simulink model "buckConverter"  (R2023a)
settings: Solver=VariableStepAuto  StartTime=0.0  StopTime=inf  RelTol=1e-3
model workspace (MAT data in the model file):
  C = Simulink.Parameter
  C.Value = 0.01
  C.DataType = 'double'
  C.Complexity = 'real'
  C.Dimensions = [1 1]
  L = Simulink.Parameter
  L.Value = 0.01
  L.DataType = 'double'
  L.Complexity = 'real'
  L.Dimensions = [1 1]
  R = Simulink.Parameter
  R.Value = 10
  R.DataType = 'double'
  R.Complexity = 'real'
  R.Dimensions = [1 1]
  Vin = Simulink.Parameter
  Vin.Value = 100
  Vin.DataType = 'double'
  Vin.Complexity = 'real'
  Vin.Dimensions = [1 1]
libraries: spsCurrentMeasurementLib x8, spsSeriesRLCBranchLib x6, spsVoltageMeasurementLib x4, spsMeanLib x3, spsMosfetLib x3, spsDCVoltageSourceLib x2, spsDiodeLib x1, spspowerguiLib x1
settings Model: Creator=User  LastModifiedBy=User
settings DebuggingCC: UnconnectedInputMsg=warning  UnconnectedOutputMsg=warning  UnconnectedLineMsg=warning
settings ModelReferenceCC: EnableRefExpFcnMdlSchedulingChecks=on
settings RTWCC: DLArmComputeVersion=19.05

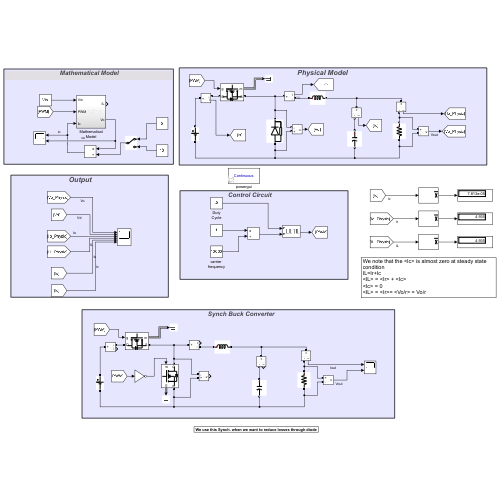
[thumbnail: Simulink's stored preview of the top-level diagram]
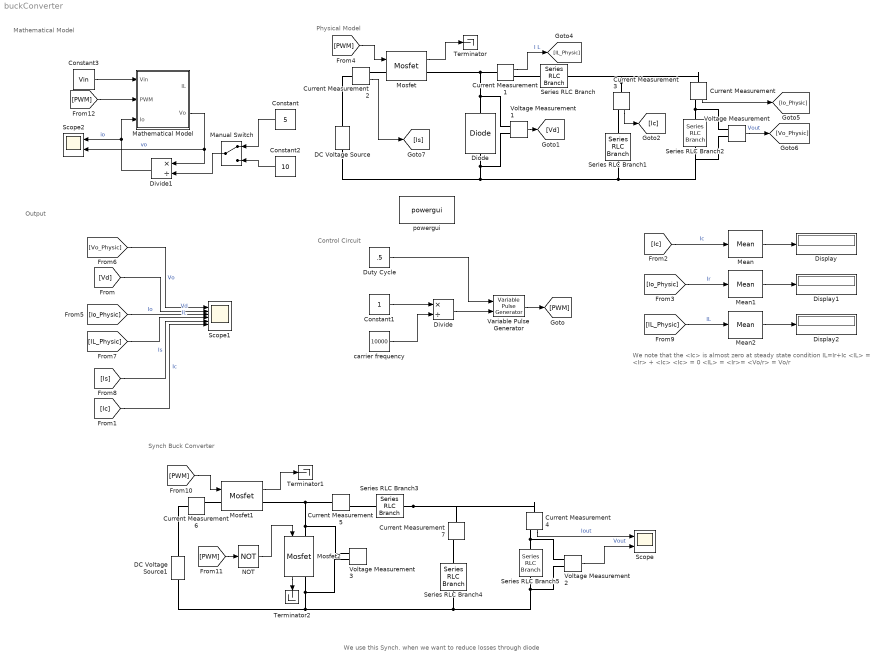
== system buckConverter ==
  note: We use this Synch. when we want to reduce losses through diode
  note: Synch Buck Converter
  note: We note that the <Ic> is almost zero at steady state condition
      | IL=Ir+Ic
      | <IL> = <Ir> + <Ic>
      | <Ic> = 0
      | <IL> = <Ir>= <Vo/r> = Vo/r
  note: Output
  note: Mathematical Model
  note: Physical Model
  note: Control Circuit
  Constant : Constant  Value=5
  Constant1 : Constant
  Constant2 : Constant  Value=10
  Constant3 : Constant  Value=Vin
  Current Measurement{,1..7} (8 alike) : spsCurrentMeasurementLib/Current Measurement  PhasorSimulation=off  OutputType=Complex  PSBequivalent=0
  DC Voltage Source : spsDCVoltageSourceLib/DC Voltage Source  Amplitude=Vin  Measurements=None
  DC Voltage Source1 : spsDCVoltageSourceLib/DC Voltage Source  Amplitude=Vin  Measurements=None
  Diode : spsDiodeLib/Diode  Ron=0.001  Lon=0  Vf=0.8  IC=0  UseSnubber=0  Rs=500  Cs=250e-9  Measurements=off
  Display : Display
  Display1 : Display
  Display2 : Display
  Divide : Product  Inputs=*/
  Divide1 : Product  Inputs=*/
  Duty Cycle : Constant  Value=.5
  Manual Switch : ManualSwitch
  Mathematical Model : Subsystem
  Mean : spsMeanLib/Mean  Freq=60  Vinit=0  Ts=0
  Mean1 : spsMeanLib/Mean  Freq=60  Vinit=0  Ts=0
  Mean2 : spsMeanLib/Mean  Freq=60  Vinit=0  Ts=0
  Mosfet : spsMosfetLib/Mosfet  Ron=0.1  Lon=0  Rd=0.01  Vfd=0  IC=0  Rs=1e5  Cs=inf  Measurements=on
  Mosfet1 : spsMosfetLib/Mosfet  Ron=0.1  Lon=0  Rd=0.01  Vfd=0  IC=0  Rs=1e5  Cs=inf  Measurements=on
  Mosfet2 : spsMosfetLib/Mosfet  Ron=0.1  Lon=0  Rd=0.01  Vfd=0  IC=0  Rs=1e5  Cs=inf  Measurements=on
  NOT : Logic  Operator=NOT  IconShape=distinctive  AllPortsSameDT=off  OutDataTypeStr=boolean
  Scope : Scope  NumInputPorts=2
  Scope1 : Scope  NumInputPorts=6
  Scope2 : Scope  NumInputPorts=2
  Series RLC Branch : spsSeriesRLCBranchLib/Series RLC Branch  LConnTagsString=__new0  RConnTagsString=__new0  BranchType=L  Resistance=1  Inductance=L  SetiL0=off  InitialCurrent=0  Capacitance=1e-6  Setx0=off  InitialVoltage=0  Measurements=None
  Series RLC Branch1 : spsSeriesRLCBranchLib/Series RLC Branch  LConnTagsString=__new0  RConnTagsString=__new0  BranchType=C  Resistance=1  Inductance=1e-3  SetiL0=off  InitialCurrent=0  Capacitance=C  Setx0=off  InitialVoltage=0  Measurements=None
  Series RLC Branch2 : spsSeriesRLCBranchLib/Series RLC Branch  LConnTagsString=__new0  RConnTagsString=__new0  BranchType=R  Resistance=R  Inductance=1e-3  SetiL0=off  InitialCurrent=0  Capacitance=1e-6  Setx0=off  InitialVoltage=0  Measurements=None
  Series RLC Branch3 : spsSeriesRLCBranchLib/Series RLC Branch  LConnTagsString=__new0  RConnTagsString=__new0  BranchType=L  Resistance=1  Inductance=L  SetiL0=off  InitialCurrent=0  Capacitance=1e-6  Setx0=off  InitialVoltage=0  Measurements=None
  Series RLC Branch4 : spsSeriesRLCBranchLib/Series RLC Branch  LConnTagsString=__new0  RConnTagsString=__new0  BranchType=C  Resistance=1  Inductance=1e-3  SetiL0=off  InitialCurrent=0  Capacitance=C  Setx0=off  InitialVoltage=0  Measurements=None
  Series RLC Branch5 : spsSeriesRLCBranchLib/Series RLC Branch  LConnTagsString=__new0  RConnTagsString=__new0  BranchType=R  Resistance=R  Inductance=1e-3  SetiL0=off  InitialCurrent=0  Capacitance=1e-6  Setx0=off  InitialVoltage=0  Measurements=None
  Terminator : Terminator
  Terminator1 : Terminator
  Terminator2 : Terminator
  Variable Pulse Generator : VariablePulseGenerator  SampleTime=0.1
  Voltage Measurement{,1..3} (4 alike) : spsVoltageMeasurementLib/Voltage Measurement  PhasorSimulation=off  OutputType=Complex  PSBequivalent=0
  carrier frequency : Constant  Value=10000
  powergui : spspowerguiLib/powergui  Priority=1  SimulationMode=Continuous  SampleTime=50e-6  frequency=60  Iterations=50  frequencyindice=0  Pbase=100e6  ErrMax=1e-4  UnitsV=kV  UnitsW=MW  buscounter=0  FunctionMessages=off  echomessages=off  EnableUseOfTLC=off  CurrentSourceSwitches=off  DisableSnubberDevices=off  DisableRonSwitches=off  DisableVfSwitches=off  DisplayEquations=off  AutomaticDiscreteSolvers=off  SolverType=Tustin/Backward Euler (TBE)  Interpol=off  ExternalGateDelay=off  methode=off  Ts=100  x0status=blocks  SPID=on  SwTol=0  HookPort=off  NonlinearTolerance=1e-4  nMaxIteration=100  ContinueOnMaxIteration=off  RestoreLinks=warning  ResistiveCurrentMeasurement=off  Frange=[0:2:500]  Ylog=off  Xlog=on  ShowGrid=off  save=off  variable=ZData  structure=0  ZoomFFT=off  StartTime=0.0  cycles=1  DisplayStyle=1  fundamental=60  FreqAxis=off  MaxFrequency=1000  frequencyindicesteady=1  RmsSteady=1  display=off
  wires:
  Variable Pulse Generator/1 -> [PWM]
  Duty Cycle/1 -> Variable Pulse Generator/1
  Divide/1 -> Variable Pulse Generator/2
  Constant1/1 -> Divide/1
  carrier frequency/1 -> Divide/2
  Mathematical Model/2(Vo) -> Divide1/1, Scope2/2  "vo"
  Divide1/1 -> Mathematical Model/3(Io), Scope2/1  "io"
  [Io_Physic] -> Scope1/3  "Io"
  [IL_Physic] -> Scope1/4  "IL"
  Current Measurement1/1 -> [IL_Physic]  "I L"
  Current Measurement/1 -> [Io_Physic]
  Voltage Measurement/1 -> [Vo_Physic]  "Vout"
  [Vo_Physic] -> Scope1/1  "Vo"
  [PWM] -> Mosfet/1
  Mosfet/1 -> Terminator/1
  Current Measurement2/1 -> [Is]
  [Is] -> Scope1/5  "Is"
  Voltage Measurement1/1 -> [Vd]
  [Vd] -> Scope1/2  "Vd"
  Current Measurement3/1 -> [Ic]
  [Ic] -> Scope1/6  "Ic"
  Mean/1 -> Display/1
  [Ic] -> Mean/1  "Ic"
  [Io_Physic] -> Mean1/1  "Ir"
  Mean1/1 -> Display1/1
  Mean2/1 -> Display2/1
  [IL_Physic] -> Mean2/1  "IL"
  Mosfet1/1 -> Terminator1/1
  [PWM] -> Mosfet1/1
  Voltage Measurement2/1 -> Scope/2  "Vout"
  Current Measurement4/1 -> Scope/1  "Iout"
  [PWM] -> NOT/1
  NOT/1 -> Mosfet2/1
  Mosfet2/1 -> Terminator2/1
  Constant/1 -> Manual Switch/1
  Manual Switch/1 -> Divide1/2
  Constant2/1 -> Manual Switch/2
  Constant3/1 -> Mathematical Model/1(Vin)
  [PWM] -> Mathematical Model/2(PWM)
  connections:
  DC Voltage Source/LConn1 -- Voltage Measurement/LConn2 -- Series RLC Branch2/RConn1 -- Series RLC Branch1/RConn1 -- Voltage Measurement1/LConn1 -- Diode/LConn1
  Series RLC Branch2/LConn1 -- Voltage Measurement/LConn1 -- Current Measurement/RConn1
  Series RLC Branch1/LConn1 -- Current Measurement3/RConn1
  Series RLC Branch/LConn1 -- Current Measurement1/RConn1
  Diode/RConn1 -- Voltage Measurement1/LConn2 -- Mosfet/RConn1 -- Current Measurement1/LConn1
  Current Measurement2/LConn1 -- DC Voltage Source/RConn1
  Mosfet/LConn1 -- Current Measurement2/RConn1
  Current Measurement3/LConn1 -- Series RLC Branch/RConn1 -- Current Measurement/LConn1
  Voltage Measurement2/LConn2 -- Series RLC Branch5/RConn1 -- Series RLC Branch4/RConn1 -- DC Voltage Source1/LConn1 -- Voltage Measurement3/LConn1 -- Mosfet2/RConn1
  Series RLC Branch5/LConn1 -- Current Measurement4/RConn1 -- Voltage Measurement2/LConn1
  Voltage Measurement3/LConn2 -- Current Measurement5/LConn1 -- Mosfet1/RConn1 -- Mosfet2/LConn1
  Series RLC Branch3/RConn1 -- Current Measurement7/LConn1 -- Current Measurement4/LConn1
  Mosfet1/LConn1 -- Current Measurement6/RConn1
  Series RLC Branch3/LConn1 -- Current Measurement5/RConn1
  Series RLC Branch4/LConn1 -- Current Measurement7/RConn1
  Current Measurement6/LConn1 -- DC Voltage Source1/RConn1

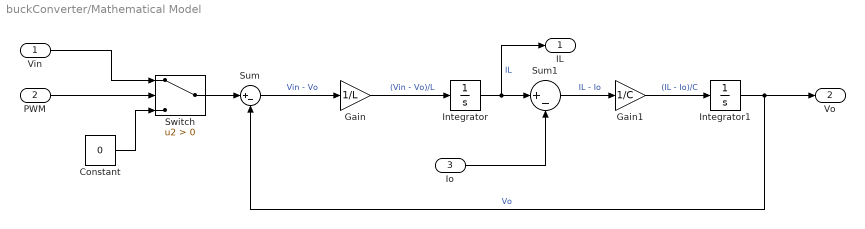
== system buckConverter/Mathematical Model ==
  Vin : Inport
  PWM : Inport  Port=2
  Io : Inport  Port=3
  Constant : Constant  Value=0
  Gain : Gain  Gain=1/L
  Gain1 : Gain  Gain=1/C
  Integrator : Integrator
  Integrator1 : Integrator
  Sum : Sum  Inputs=|+-
  Sum1 : Sum  Inputs=|+-
  Switch : Switch  Criteria=u2 > Threshold  SaturateOnIntegerOverflow=off  InputSameDT=off
  IL : Outport
  Vo : Outport  Port=2
  wires:
  Integrator/1 -> IL/1, Sum1/1  "IL"
  Vin/1 -> Switch/1
  Gain1/1 -> Integrator1/1  "(IL - Io)/C"
  Integrator1/1 -> Vo/1, Sum/2  "Vo"
  PWM/1 -> Switch/2
  Sum/1 -> Gain/1  "Vin - Vo"
  Switch/1 -> Sum/1
  Constant/1 -> Switch/3
  Gain/1 -> Integrator/1  "(Vin - Vo)/L"
  Sum1/1 -> Gain1/1  "IL - Io"
  Io/1 -> Sum1/2
